simulink model "EKF_noBias_Testing"  (R2020b)
settings: Solver=FixedStepAuto  StartTime=0.0  StopTime=sim_constants.simulation_time  FixedStep=sim_constants.time_step  RelTol=1e-3
values from neighbouring files (symbols this model uses):
  B_ECI = B_ECI    [EKF_nobias_runtest.m]    (also in EKF_runtest.m = B_ECI.Data)
  B_meas = B_meas    [EKF_nobias_runtest.m]    (also in EKF_runtest.m = B_meas.Data)
  M = M_perturbations.Data    [EKF_nobias_runtest.m]    (also in EKF_runtest.m)
  S_ECI = S_ECI.Data    [EKF_nobias_runtest.m]    (also in EKF_runtest.m)
  Sazel_meas = Sazel_meas.Data    [EKF_nobias_runtest.m]    (also in EKF_runtest.m)
  w_meas = squeeze(w_meas.Data).'    [EKF_nobias_runtest.m]    (also in EKF_runtest.m)
undefined symbols (not defined in the file or in its folder): sim_constants
settings Model: Creator=newpo  LastModifiedBy=newpo
settings DataIOCC: ReturnWorkspaceOutputs=off

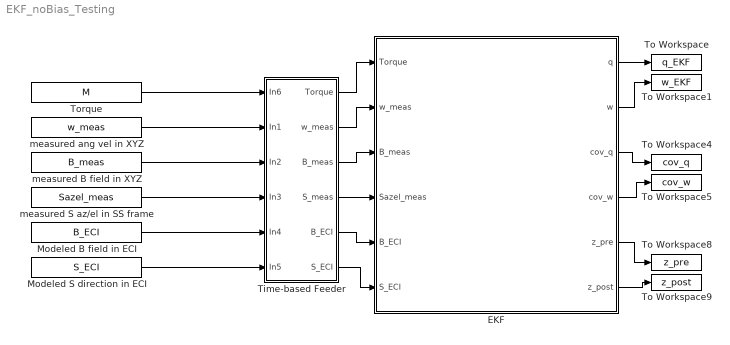
== system EKF_noBias_Testing ==
  EKF : Subsystem
  Modeled B field in ECI : Constant  Value=B_ECI
  Modeled S direction in ECI : Constant  Value=S_ECI
  Time-based Feeder : Subsystem
  To Workspace : ToWorkspace  VariableName=q_EKF  SaveFormat=Timeseries  SampleTime=-1
  To Workspace1 : ToWorkspace  VariableName=w_EKF  SaveFormat=Timeseries  SampleTime=-1
  To Workspace4 : ToWorkspace  VariableName=cov_q  SaveFormat=Timeseries  SampleTime=-1
  To Workspace5 : ToWorkspace  VariableName=cov_w  SaveFormat=Timeseries  SampleTime=-1
  To Workspace8 : ToWorkspace  VariableName=z_pre  SaveFormat=Timeseries  SampleTime=-1
  To Workspace9 : ToWorkspace  VariableName=z_post  SaveFormat=Timeseries  SampleTime=-1
  "Torque " : Constant  Value=M
  measured B field in XYZ : Constant  Value=B_meas
  measured S az/el in SS frame : Constant  Value=Sazel_meas
  measured ang vel in XYZ : Constant  Value=w_meas
  wires:
  measured ang vel in XYZ/1 -> Time-based Feeder/2(In1)
  measured B field in XYZ/1 -> Time-based Feeder/3(In2)
  measured S az/el in SS frame/1 -> Time-based Feeder/4(In3)
  Modeled B field in ECI/1 -> Time-based Feeder/5(In4)
  Modeled S direction in ECI/1 -> Time-based Feeder/6(In5)
  EKF/1(q) -> To Workspace/1
  EKF/2(w) -> To Workspace1/1
  EKF/3(cov_q) -> To Workspace4/1
  EKF/4(cov_w) -> To Workspace5/1
  EKF/5(z_pre) -> To Workspace8/1
  EKF/6(z_post) -> To Workspace9/1
  "Torque "/1 -> Time-based Feeder/1(In6)
  Time-based Feeder/1(Torque) -> EKF/1(Torque)
  Time-based Feeder/2(w_meas) -> EKF/2(w_meas)
  Time-based Feeder/3(B_meas) -> EKF/3(B_meas)
  Time-based Feeder/4(S_meas) -> EKF/4(Sazel_meas)
  Time-based Feeder/5(B_ECI) -> EKF/5(B_ECI)
  Time-based Feeder/6(S_ECI) -> EKF/6(S_ECI)

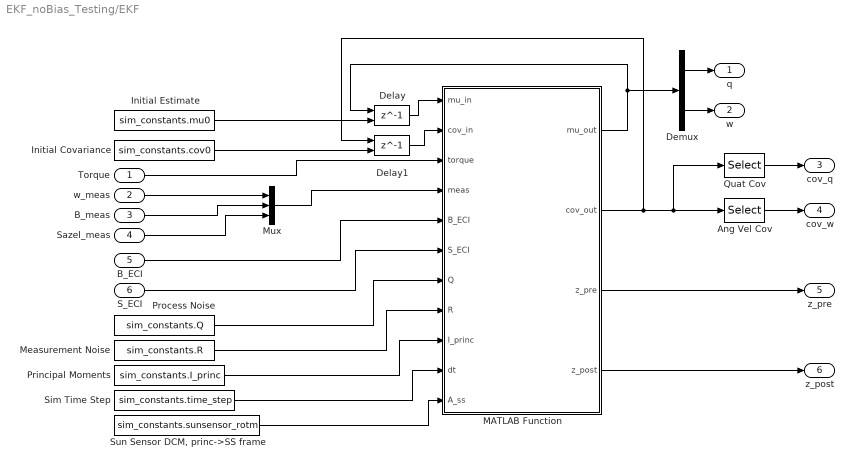
== system EKF_noBias_Testing/EKF ==
  Torque : Inport
  w_meas : Inport  Port=2
  B_meas : Inport  Port=3
  Sazel_meas : Inport  Port=4
  B_ECI : Inport  Port=5
  S_ECI : Inport  Port=6
  Ang Vel Cov : Selector  NumberOfDimensions=2  InputPortWidth=3  IndexOptions=Index vector (dialog),Index vector (dialog)  Indices=5:7,5:7  OutputSizes=1,1
  Delay : Delay  DelayLength=1  InitialConditionSource=Input port  InitialCondition=0
      settings: InputPortMap=u0,p4
  Delay1 : Delay  DelayLength=1  InitialConditionSource=Input port  InitialCondition=0
      settings: InputPortMap=u0,p4
  Demux : Demux  Outputs=[4, 3]
  Initial Covariance : Constant  Value=sim_constants.cov0
  Initial Estimate : Constant  Value=sim_constants.mu0
  MATLAB Function : MATLAB Function  TreatAsAtomicUnit=on
  Measurement Noise : Constant  Value=sim_constants.R
  Mux : Mux  Inputs=3
  Principal Moments : Constant  Value=sim_constants.I_princ
  Process Noise : Constant  Value=sim_constants.Q
  Quat Cov : Selector  NumberOfDimensions=2  InputPortWidth=3  IndexOptions=Index vector (dialog),Index vector (dialog)  Indices=1:4,1:4  OutputSizes=1,1
  Sim Time Step : Constant  Value=sim_constants.time_step
  "Sun Sensor DCM, princ->SS frame" : Constant  Value=sim_constants.sunsensor_rotm
  q : Outport
  w : Outport  Port=2
  cov_q : Outport  Port=3
  cov_w : Outport  Port=4
  z_pre : Outport  Port=5
  z_post : Outport  Port=6
  wires:
  MATLAB Function/2(cov_out) -> Delay1/1, Quat Cov/1, Ang Vel Cov/1
  Torque/1 -> MATLAB Function/3(torque)
  w_meas/1 -> Mux/1
  B_meas/1 -> Mux/2
  Sazel_meas/1 -> Mux/3
  Mux/1 -> MATLAB Function/4(meas)
  B_ECI/1 -> MATLAB Function/5(B_ECI)
  S_ECI/1 -> MATLAB Function/6(S_ECI)
  Process Noise/1 -> MATLAB Function/7(Q)
  Measurement Noise/1 -> MATLAB Function/8(R)
  Principal Moments/1 -> MATLAB Function/9(I_princ)
  Sim Time Step/1 -> MATLAB Function/10(dt)
  Demux/1 -> q/1
  Demux/2 -> w/1
  Ang Vel Cov/1 -> cov_w/1
  Quat Cov/1 -> cov_q/1
  MATLAB Function/3(z_pre) -> z_pre/1
  MATLAB Function/4(z_post) -> z_post/1
  Delay/1 -> MATLAB Function/1(mu_in)
  Delay1/1 -> MATLAB Function/2(cov_in)
  Initial Estimate/1 -> Delay/2
  Initial Covariance/1 -> Delay1/2
  MATLAB Function/1(mu_out) -> Delay/1, Demux/1
  "Sun Sensor DCM, princ->SS frame"/1 -> MATLAB Function/11(A_ss)

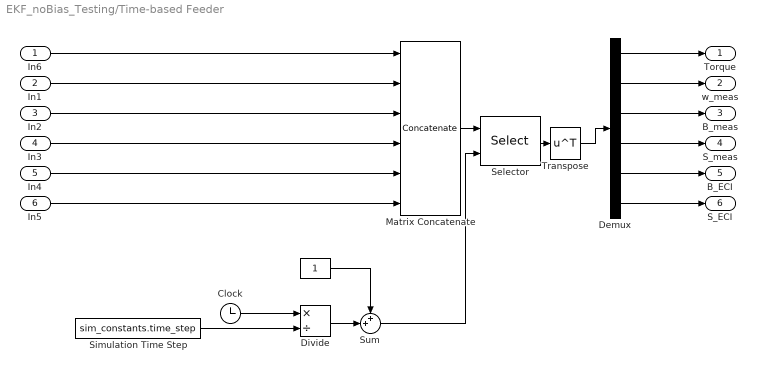
== system EKF_noBias_Testing/Time-based Feeder ==
  In6 : Inport
  In1 : Inport  Port=2
  In2 : Inport  Port=3
  In3 : Inport  Port=4
  In4 : Inport  Port=5
  In5 : Inport  Port=6
  " " : Constant
  Clock : Clock
  Demux : Demux  Outputs=[3 3 3 2 3 3]
  Divide : Product  Inputs=*/  OutDataTypeStr=int32
  Matrix Concatenate : Concatenate  NumInputs=6  Mode=Multidimensional array  ConcatenateDimension=2
  Selector : Selector  NumberOfDimensions=2  InputPortWidth=3  IndexOptions=Index vector (port),Index vector (dialog)  Indices=[1 3],-1  OutputSizes=1,1
  Simulation Time Step : Constant  Value=sim_constants.time_step
  Sum : Sum  Inputs=++|
  Transpose : Math  Operator=transpose  SaturateOnIntegerOverflow=on
  Torque : Outport
  w_meas : Outport  Port=2
  B_meas : Outport  Port=3
  S_meas : Outport  Port=4
  B_ECI : Outport  Port=5
  S_ECI : Outport  Port=6
  wires:
  Divide/1 -> Sum/2
  In5/1 -> Matrix Concatenate/6
  Selector/1 -> Transpose/1
  Sum/1 -> Selector/2
  Matrix Concatenate/1 -> Selector/1
  Transpose/1 -> Demux/1
  Clock/1 -> Divide/1
  In2/1 -> Matrix Concatenate/3
  Simulation Time Step/1 -> Divide/2
  " "/1 -> Sum/1
  Demux/1 -> Torque/1
  Demux/4 -> S_meas/1
  In1/1 -> Matrix Concatenate/2
  Demux/3 -> B_meas/1
  Demux/5 -> B_ECI/1
  In4/1 -> Matrix Concatenate/5
  In3/1 -> Matrix Concatenate/4
  Demux/2 -> w_meas/1
  In6/1 -> Matrix Concatenate/1
  Demux/6 -> S_ECI/1

== matlab function EKF_noBias_Testing/EKF/MATLAB Function ==
  data: mu_in input; mu_out output; cov_in input; torque input; meas input; B_ECI input; S_ECI input; Q input; R input; I_princ input; dt input; cov_out output; z_pre output; z_post output; A_ss input
%% satEKF
% Extended Kalman filter for satellite attitude state estimation.
% mu_in : the current estimated state mean, in the form
%           (q, w, bw, bB, bS)^T
%           where q is the quaternion, w is the principal axes angular
%           velocity, bw is the gyroscopic sensor bias, bB is the magnetic
%           sensor bias, and bS is the azimuth/elevation sun sensor bias.
% cov_in : the current covariance matrix
% torque : the input torque to the system at the current time step
% meas : the measurement of the current state
% B_ECI : the modeled magnetic field vector in inertial coordinates at current time
% S_ECI: the modeled sun-pointing vector in intertial coordinates at current time 
% Q : the process noise matrix
% R : the measurement noise matrix
% I_princ : the principal moments of inertia corresponding to principal XYZ
% dt : the time step
% A_ss : the rotation from principal axes to sun sensor frame
function [mu_out, cov_out, z_pre, z_post] = satEKF_nobias(mu_in, cov_in, torque, meas, B_ECI, S_ECI, Q, R, I_princ, dt, A_ss)
    q = mu_in(1:4); % quaternion
    q = q/norm(q);
    w = mu_in(5:7); % angular velocity in princ
    
    At = A(q,w,I_princ,dt);
    %% Predict - use non-linear function to predict mean, linearized info for cov
    mu_p = f(mu_in,torque,I_princ,dt); % get predicted state from non-linear eq
    cov_p = At*cov_in*(At.') + Q;
    A_p = q2A(mu_p(1:4)/norm(mu_p(1:4))); % get rotation matrix of predicted state
    meas_p = g(mu_p,A_p*B_ECI,A_p*S_ECI,A_ss); % predicted measurement
    z_pre = z(meas, meas_p); % pre-fit residual (diff between real and predicted)
    %% Update - use predicted states to compute Kalman gain and final update
    % Update state using sensitivity matrix
    q_p = mu_p(1:4)/norm(mu_p(1:4));
    Ct = C(q_p,q2A(q_p),B_ECI,S_ECI,A_ss); % Sensitivity matrix
    K = cov_p*(Ct.')/(Ct*cov_p*(Ct.') + R) ; % Kalman Gain
    mu_out = mu_p + K*z_pre;
    T = (eye(15) - K*Ct);
    cov_out = T*cov_p*(T.') + K*R*(K.');
    A_f = q2A(mu_out(1:4)/norm(mu_out(1:4)));
    z_post = z(meas, g(mu_out,A_f*B_ECI,A_f*S_ECI,A_ss));  % post-fit residual (diff between real and estimated)
end
% Helper Functions
    function O = Omega(w)
        % Returns Omega(w), the rate relation such that dw/dt = 0.5*Omega*q
        O = [0 w(3) -w(2) w(1);
             -w(3) 0 w(1) w(2);
             w(2) -w(1) 0 w(3);
             -w(1) -w(2) -w(3) 0];
    end
    function L = Lambda(q)
        % Returns Lambda(q), the rate relation such that dw/dt = 0.5*Lambda*w
        L = [q(4) -q(3) q(2);
             q(3) q(4) -q(1);
             -q(2) q(1) q(4);
             -q(1) -q(2) -q(3) ];
    end
    function D = Delta(w,I)
        % Returns Delta(w), the partial derivative of the Euler equations
        % wrt angular velocity.
        D = [0 (I(2)-I(3))/I(1)*w(3) (I(2)-I(3))/I(1)*w(2);
             (I(3)-I(1))/I(2)*w(3) 0 (I(3)-I(1))/I(2)*w(1);
             (I(1)-I(2))/I(3)*w(2) (I(1)-I(2))/I(3)*w(1) 0 ];
    end
    function G = Gamma(q,V)
        % Returns Gamma(q,V), the partial derivative of A(q)*V wrt to the
        % quaternion, for some vector V in ECI.
        q = q/norm(q);
        qvec = q(1:3);
        a = [-q(2);q(1);-q(4)];
        b = [-q(3);q(4);q(1)];
        c = [q(4); q(3); -q(2)];
        G = 2*[dot(qvec,V) dot(a,V) dot(b,V) dot(c,V);
               dot(-a,V) dot(qvec,V) dot(-c,V) dot(b,V);
               dot(-b,V) dot(c,V) dot(qvec,V) dot(-a,V) ];
    end
    function Mt = M(S)
        Mt = [atan2(S(2),S(1)); acos(S(3))];
    end
    function Mt = Mtilde(S)
        S12 = S(1)^2 + S(2)^2;
        Mt = [-S(2)/S12 S(1)/S12 0; 0 0 -1/sqrt(1-S(3)^2)];
    end
    function xout = f(x,torque,I,dt)
        % Dynamics function such that x_{t+1} = f(x_t, u_t)
        q = x(1:4);
        w = x(5:7);
        s = eye(7); 
        normq = norm(q);
        s(1:4,1:4) = eye(4)/normq;
        xout = s*(x + dt*[0.5*Omega(w)*q ; (torque - cross(w,I.*w))./I]);
    end
    function At = A(q,w,I,dt)
        % Jacobian of dynamics
        normq = norm(q);
        q = q/normq;
        s = eye(7); 
        b = diag((normq^2)*ones(4,1)-(q.^2)); % b = d/dq of (q/norm(q))
        b(1,2:4) = -q(2:4).' * q(1) ;
        b(2,[1 3 4]) = -q([1 3 4]).' * q(2) ;
        b(3,[1 2 4]) = -q([1 2 4]).' * q(3) ;
        b(2,[1 2 3]) = -q([1 2 3]).' * q(4) ;
        b = b/(normq^3);
        s(1:4,1:4) = b;
        At = s + dt*[0.5*Omega(w).*b 0.5*Lambda(q)/normq;
              zeros(3,4) Delta(w,I) ];
    end
    function y = g(x,B_XYZ,S_XYZ,A_ss)
        % Measurement function such that y_t = g(x_t,u_t)
        % A is the computed rotation matrix taken from the first four
        % elements of x
        y = zeros(8,1);
        y(1:3) = x(5:7); % angular velocity measurement, w/ bias
        y(4:6) = B_XYZ ; % magnetic field strength in XYZ, w/ bias
        y(7:8) = M(A_ss*S_XYZ); % sun az/el in sensor frame w/ bias
        y(7) = mod(y(7),2*pi); % wrap azimuth to 2*pi
        % Limit to elevation to (-90, 90)
        if y(8) < -pi/2
            y(8) = -pi - y(8);
            y(7) = mod(y(7) + pi, 2*pi);
        elseif y(8) > pi/2 
            y(8) = pi - y(8);
            y(7) = mod(y(7) + pi, 2*pi);
        end
    end
    function Ct = C(q,Aq,B_ECI,S_ECI,A_ss)
        S_xyz = Aq*S_ECI;
        Ct = [zeros(3,4) eye(3);
              Gamma(q,B_ECI) zeros(3);
              Mtilde(A_ss*S_xyz)*A_ss*Gamma(q,S_ECI) zeros(2,3)];
    end
    function zt = z(y, g)
        zt = y-g;
        azy = y(7); ely = y(8);
        azg = g(7); elg = g(8);
        % check if azimuth is near the turn-over point 2*pi->0
        if azy < pi/2 && azg > 3*pi/2
           azg = azg - 2*pi;
        elseif azy > 3*pi/2 && azg < pi/2
           azy = azy - 2*pi;
        end
        % check that azimuths aren't near-opposite, if so, flip
        if abs(azy-azg) > pi/0
            azg = mod(azg+pi, 2*pi); % flip azg
            if elg > 0
               elg = pi - elg;
            else
               elg = -pi - elg;
            end
        end
        zt(7:8) = [azy-azg; ely-elg];
    end
